simulink library "Valve_Thermostatic"  (R2018b)
settings: Solver=ode45  StartTime=0.0  StopTime=10.0  RelTol=1e-3  EnableMultiTasking=on
undefined symbols (not defined in the file): linear
libraries: carnot x2
settings Model: Creator=lena.frank  LastModifiedBy=P41573
settings DataIOCC: LimitDataPoints=on  SaveFormat=Array  SignalLoggingSaveFormat=ModelDataLogs
settings OptimizationCC: ExpressionDepthLimit=2147483647  LifeSpan=inf
settings DebuggingCC: UnderspecifiedInitializationDetection=Classic  MergeDetectMultiDrivingBlocksExec=none  SolverPrmCheckMsg=warning  FcnCallInpInsideContextMsg=warning  StateNameClashWarn=warning  SFUnexpectedBacktrackingDiag=warning  SFNoUnconditionalDefaultTransitionDiag=warning  SFExecutionAtInitializationDiag=none
settings HardwareCC: ProdBitPerPointer=32  ProdBitPerSizeT=32  ProdBitPerPtrDiffT=32  ProdLargestAtomicFloat=None  ProdIntDivRoundTo=Undefined  ProdEndianess=Unspecified  ProdWordSize=32  ProdHWDeviceType=32-bit Generic
settings ModelReferenceCC: PropagateSignalLabelsOutOfModel=off
settings SFSimCC: SimUseLocalCustomCode=off
settings RTWCC: RTWUseLocalCustomCode=off
settings CodeAppCC: StateflowObjectComments=on
settings GRTTargetCC: TargetLangStandard=C89/C90 (ANSI)  GeneratePreprocessorConditionals=Disable all  CombineOutputUpdateFcns=off  GRTInterface=on
settings ConfigComp: CovMetricSettings=dw  CovHtmlReporting=on  CovSaveCumulativeToWorkspaceVar=on  CovSaveSingleToWorkspaceVar=on  CovExternalEMLEnable=off

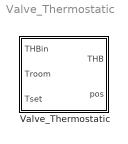
== system Valve_Thermostatic ==
  Valve_Thermostatic : Subsystem  mask(thermostatic valve){p=4, op=0.5, bl=0.2, ts=1, dt_V=1, ART=linear, kvs=2, psi_0=0.04}
      mask prompts: p "Proportional range in K"; op "Operation point (valve position at set temperature)"; bl "Hysteresis or play in K"; ts "First order hold for temperature sensor in s"; dt_V "Valve running time in s"; ART "Valve characteristic"; kvs "Kvs: flow coefficient of the open valve in m³/h"; psi_0 "Psi_0: relative flow coefficient Kv/Kvs of the closed valve"
      mask help: Thermostatic valve for a radiator.
      mask Help: web(fullfile(path_carnot('help'),'Valve_Thermostatic.html'),'-helpbrowser')
      mask TypeOptions p: Thermostat_Proportional/p
      mask TypeOptions op: Thermostat_Proportional/op
      mask TypeOptions bl: Thermostat_Proportional/bl
      mask TypeOptions ts: Thermostat_Proportional/ts
      mask TypeOptions dt_V: Valve/dt_V
      mask TypeOptions ART: Valve/vtyp
      mask TypeOptions kvs: Valve/kvs
      mask TypeOptions psi_0: Valve/psi_0
      mask DialogControl ParameterTabVar0 Prompt: Thermostat
      mask DialogControl ParameterTabVar01 Prompt: Hydraulic
      mask Display:
      | plot(-20,-20,120,120,[10,90,90,10,10],[50,0,50,0,50],...
      |     [50,50],[50,25],...
      |     [40,30,30,40,60,70,70,60,40],[50,60,80,90,90,80,60,50,50],...
      |     [60,40],[80,80],[50,50],[60,80])

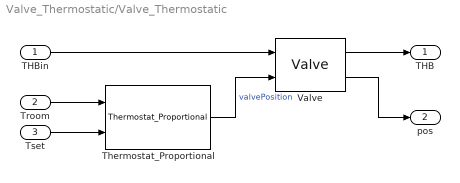
== system Valve_Thermostatic/Valve_Thermostatic ==
  THBin : Inport
  Troom : Inport  Port=2
  Tset : Inport  Port=3
  Thermostat_Proportional : carnot/Control/Thermostat_Proportional  op=op  bl=bl  p=p  ts=ts
      settings: SourceProductName=Carnot
  Valve : carnot/Hydraulics/Valve  vtyp=linear  psi_0=psi_0  kvs=kvs  dt_V=dt_V
      settings: SourceProductName=Carnot
  THB : Outport
  pos : Outport  Port=2
  wires:
  Valve/2 -> pos/1
  Thermostat_Proportional/1 -> Valve/2  "valvePosition"
  THBin/1 -> Valve/1
  Tset/1 -> Thermostat_Proportional/2
  Troom/1 -> Thermostat_Proportional/1
  Valve/1 -> THB/1
